simulink model "virtual_aero2_quick_start"  (R2021a)
settings: Solver=ode1  StartTime=0.0  StopTime=inf  FixedStep=0.002  RelTol=1e-3
undefined symbols (not defined in the file): HIL, qc_get_step_size
libraries: quarc_library x7
settings Model: Creator=MLevis  LastModifiedBy=MLevis
settings DataIOCC: ReturnWorkspaceOutputs=off

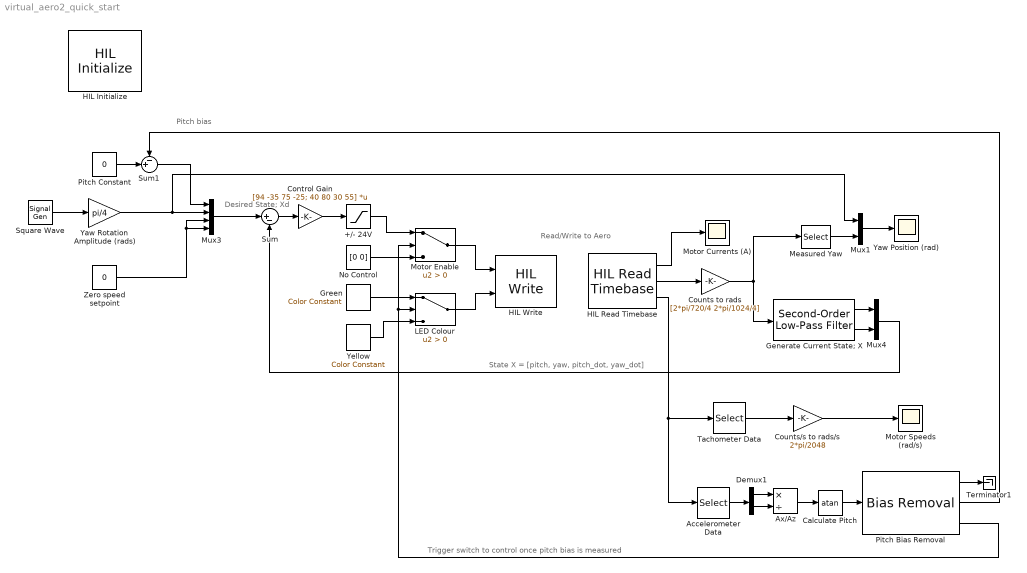
== system virtual_aero2_quick_start ==
  note: Trigger switch to control once pitch bias is measured
  note: Pitch bias
  note: Read/Write to Aero
  note: Desired State; Xd
  note: State X = [pitch, yaw, pitch_dot, yaw_dot]
  +/- 24V : Saturate  UpperLimit=24  LowerLimit=-24
  Accelerometer Data : Selector  InputPortWidth=4  IndexOptions=Index vector (dialog)  Indices=[1 2]  OutputSizes=1
  Ax/Az : Product  Inputs=*/
  Calculate Pitch : Trigonometry  Operator=atan
  Control Gain : Gain  Gain=[94 -35 75 -25; 40 80 30 55]  Multiplication=Matrix(K*u)
  Counts to rads : Gain  Gain=[2*pi/720/4 2*pi/1024/4]
  Counts/s to rads/s : Gain  Gain=2*pi/2048
  Demux1 : Demux  Outputs=2
  Generate Current State; X : quarc_library/Continuous/Second-Order Low-Pass Filter  params_source=Internal (dialog parameters)  input_width=50  input_zeta=0.8  input_init=0
  Green : quarc_library/Sources/Signals/Color Constant  color=[0 1 0]
      settings: SourceProductName=QUARC Targets
  HIL Initialize : quarc_library/Data Acquisition/Generic/Configuration/HIL Initialize  Priority=-99  object_name=HIL-1  board_type=quanser_aero2_usb  board_number=0@tcpip://localhost:18950  board_options=""  exclusive=off  active=on  hardware_clocks=[0]  clock_modes=[]  initial_clock_frequencies=[]  set_clock_params_at_start=off  set_clock_params_at_switch_in=off  set_clock_frequencies_at_start=off  set_clock_frequencies_at_switch_in=off  analog_input_channels=[0:1]  analog_input_configurations=[]  analog_input_maximums=3  analog_input_minimums=-3  set_analog_input_params_at_start=off  set_analog_input_params_at_switch_in=off  analog_output_channels=[0:1]  analog_output_maximums=24  analog_output_minimums=-24  initial_analog_outputs=[0]  final_analog_outputs=[0]  watchdog_analog_outputs=[0]  set_analog_output_params_at_start=off  set_analog_output_params_at_switch_in=off  set_analog_outputs_at_start=on  set_analog_outputs_at_switch_in=off  set_analog_outputs_at_terminate=on  set_analog_outputs_at_switch_out=off  set_analog_outputs_on_watchdog=on  digital_input_channels=[]  digital_output_channels=[0:1]  digital_output_configuration=[]  initial_digital_outputs=[1]  final_digital_outputs=[0]  watchdog_digital_outputs=[0]  set_digital_output_params_at_start=off  set_digital_output_params_at_switch_in=off  set_digital_outputs_at_start=on  set_digital_outputs_at_switch_in=off  set_digital_outputs_at_terminate=on  set_digital_outputs_at_switch_out=off  set_digital_outputs_on_watchdog=on  encoder_channels=[0:3]  quadrature=[4]  encoder_filter_frequency=[]  initial_encoder_counts=[0]  set_encoder_params_at_start=off  set_encoder_params_at_switch_in=off  set_encoder_counts_at_start=on  set_encoder_counts_at_switch_in=off  pwm_channels=[]  pwm_modes=[]  pwm_frequency=[]  pwm_configuration=[]  pwm_alignment=[]  pwm_polarity=[]  pwm_leading_deadband=[]  pwm_trailing_deadband=[]  initial_pwm_outputs=[]  final_pwm_outputs=[]  watchdog_pwm_outputs=[]  set_pwm_params_at_start=off  set_pwm_params_at_switch_in=off  set_pwm_outputs_at_start=off  set_pwm_outputs_at_switch_in=off  set_pwm_outputs_at_terminate=off  set_pwm_outputs_at_switch_out=off  set_pwm_outputs_on_watchdog=off  other_output_channels=[11000:11002]  initial_other_outputs=[0 1 0]  final_other_outputs=[1 0 0]  watchdog_other_outputs=[0 0 1]  set_other_outputs_at_start=on  set_other_outputs_at_switch_in=off  set_other_outputs_at_terminate=on  set_other_outputs_at_switch_out=off  set_other_outputs_on_watchdog=on
  HIL Read Timebase : quarc_library/Data Acquisition/Generic/Timebases/HIL Read Timebase  object_name=HIL-1  clock=0  analog_channels=[0:1]  encoder_channels=[2:3]  digital_channels=[]  other_channels=[4000 4002 14000:14001]  active=on  vector_output=on  data_type_mode=Inherit via back propagation  encoder_data_type=double  digital_data_type=boolean  overflow_mode=Synchronize (for simulated cards only)  samples_in_buffer=max(ceil(1/qc_get_step_size), 1)
  HIL Write : quarc_library/Data Acquisition/Generic/Immediate I//O/HIL Write  object_name=HIL-1  analog_channels=[0:1]  pwm_channels=[]  digital_channels=[]  other_channels=[11000:11002]  sample_time=-1  active=on  vector_input=on
  LED Colour : Switch  Criteria=u2 > Threshold
  Measured Yaw : Selector  InputPortWidth=2  IndexOptions=Index vector (dialog)  Indices=[2]  OutputSizes=1
  Motor Currents (A) : Scope
  Motor Enable : Switch  Criteria=u2 > Threshold
  Motor Speeds (rad/s) : Scope
  Mux1 : Mux  Inputs=2
  Mux3 : Mux
  Mux4 : Mux  Inputs=2
  No Control : Constant  Value=[0 0]
  Pitch Bias Removal : quarc_library/Discrete/Bias Removal  start_time=0  end_time=1  switch_id=0  sample_time=qc_get_step_size
      settings: SourceProductName=QUARC Targets
  Pitch Constant : Constant  Value=0
  "Square Wave " : SignalGenerator  WaveForm=square  Frequency=0.05
  Sum : Sum  Inputs=|+-
  Sum1 : Sum  Inputs=-+|
  Tachometer Data : Selector  InputPortWidth=4  IndexOptions=Index vector (dialog)  Indices=[3 4]  OutputSizes=1
  Terminator1 : Terminator
  Yaw Position (rad) : Scope
  Yaw Rotation Amplitude (rads) : Gain  Gain=pi/4
  Yellow : quarc_library/Sources/Signals/Color Constant  color=[1 1 0]
      settings: SourceProductName=QUARC Targets
  Zero speed setpoint : Constant  Value=0
  wires:
  Pitch Bias Removal/3 -> Motor Enable/2, LED Colour/2
  +/- 24V/1 -> Motor Enable/1
  Pitch Bias Removal/1 -> Terminator1/1
  Measured Yaw/1 -> Mux1/2
  Generate Current State; X/1 -> Mux4/1
  No Control/1 -> Motor Enable/3
  Pitch Constant/1 -> Sum1/2
  Generate Current State; X/2 -> Mux4/2
  Zero speed setpoint/1 -> Mux3/3, Mux3/4
  Yaw Rotation Amplitude (rads)/1 -> Mux3/2, Mux1/1
  Tachometer Data/1 -> Counts/s to rads/s/1
  Calculate Pitch/1 -> Pitch Bias Removal/1
  Mux4/1 -> Sum/2
  Control Gain/1 -> +/- 24V/1
  "Square Wave "/1 -> Yaw Rotation Amplitude (rads)/1
  Sum1/1 -> Mux3/1
  HIL Read Timebase/2 -> Counts to rads/1
  Ax/Az/1 -> Calculate Pitch/1
  HIL Read Timebase/1 -> Motor Currents (A)/1
  Mux1/1 -> Yaw Position (rad)/1
  Demux1/2 -> Ax/Az/2
  Counts/s to rads/s/1 -> Motor Speeds (rad/s)/1
  Pitch Bias Removal/2 -> Sum1/1
  Sum/1 -> Control Gain/1
  Accelerometer Data/1 -> Demux1/1
  HIL Read Timebase/3 -> Accelerometer Data/1, Tachometer Data/1
  Motor Enable/1 -> HIL Write/1
  Yellow/1 -> LED Colour/3
  LED Colour/1 -> HIL Write/2
  Counts to rads/1 -> Measured Yaw/1, Generate Current State; X/1
  Green/1 -> LED Colour/1
  Demux1/1 -> Ax/Az/1
  Mux3/1 -> Sum/1
